simulink model "test55"  (R2015a)
settings: Solver=ode4  StartTime=0.0  StopTime=10  FixedStep=0.0001  RelTol=1e-3
values from neighbouring files (symbols this model uses):
  d1 = m0 + m1 + m2    (= 2.75)    [test3.m]    (also in test4.m; test5.m = 0.00498784618394)
  d2 = (m1/2 + m2) * l1    (= 0.5)    [test3.m]    (also in test4.m; test5.m = 0.00670234055869)
  d3 = m2 * l2/2    (= 0.28125)    [test3.m]    (also in test4.m; test5.m = 0.00902586221044)
  f1 = (m1/2 + m2) * l1 * g    (= 4.9)    [test3.m]    (also in test4.m; test5.m = 0.66350669926)
  f2 = m2 * l2 *g/2    (= 2.75625)    [test3.m]    (also in test4.m; test5.m = 0.891162386564)
settings Model: Creator=joseg  LastModifiedBy=joseg
settings SolverCC: AlgebraicLoopSolver=LineSearch

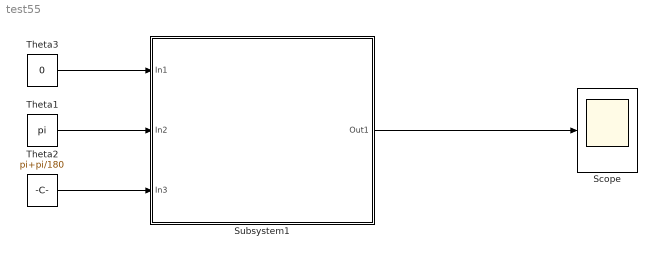
== system test55 ==
  Scope : Scope
      settings: TimeRange=14.3  YMin=-40000  YMax=5000
  Subsystem1 : Subsystem
  Theta1 : Constant  Value=pi
  Theta2 : Constant  Value=pi+pi/180
  Theta3 : Constant  Value=0
  wires:
  Theta1/1 -> Subsystem1/2(In2)
  Theta2/1 -> Subsystem1/3(In3)
  Theta3/1 -> Subsystem1/1(In1)
  Subsystem1/1(Out1) -> Scope/1

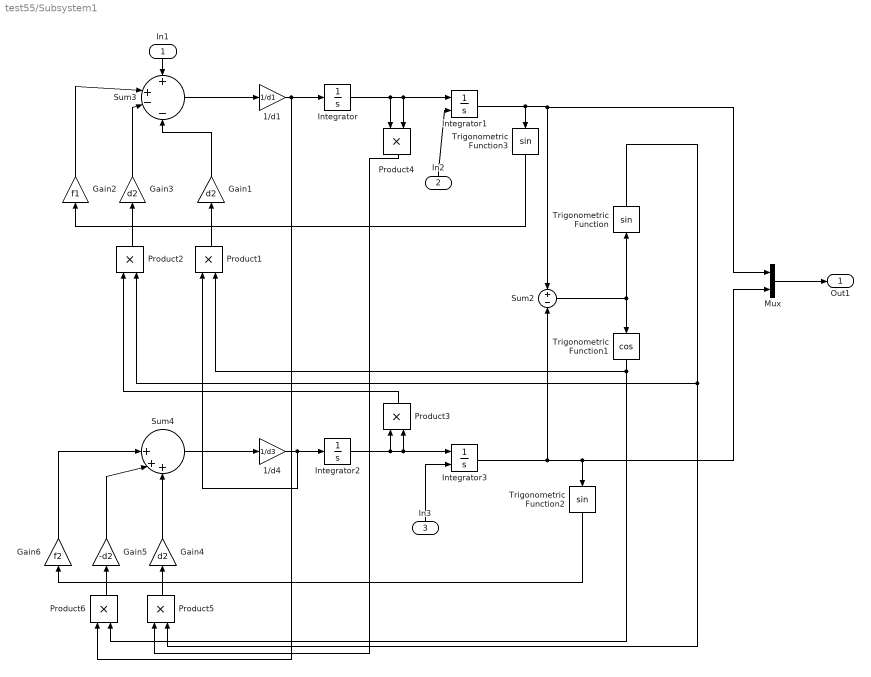
== system test55/Subsystem1 ==
  In1 : Inport
  In2 : Inport  Port=2
  In3 : Inport  Port=3
  1/d1 : Gain  Gain=1/d1
  1/d4 : Gain  Gain=1/d3
  Gain1 : Gain  Gain=d2
  Gain2 : Gain  Gain=f1
  Gain3 : Gain  Gain=d2
  Gain4 : Gain  Gain=d2
  Gain5 : Gain  Gain=-d2
  Gain6 : Gain  Gain=f2
  Integrator : Integrator
  Integrator1 : Integrator  InitialConditionSource=external
  Integrator2 : Integrator
  Integrator3 : Integrator  InitialConditionSource=external
  Mux : Mux  Inputs=2
  Product{1..6} (6 alike) : Product
  Sum2 : Sum  Inputs=+|-
  Sum3 : Sum  Inputs=+|+-|-
  Sum4 : Sum  Inputs=||+++
  Trigonometric Function : Trigonometry
  Trigonometric Function1 : Trigonometry  Operator=cos
  Trigonometric Function2 : Trigonometry
  Trigonometric Function3 : Trigonometry
  Out1 : Outport
  wires:
  Trigonometric Function/1 -> Product5/2, Product2/2
  Integrator2/1 -> Integrator3/1, Product3/2, Product3/1
  Product3/1 -> Product2/1
  Product6/1 -> Gain5/1
  Integrator/1 -> Product4/1, Product4/2, Integrator1/1
  Product5/1 -> Gain4/1
  Gain5/1 -> Sum4/2
  Trigonometric Function3/1 -> Gain2/1
  Gain4/1 -> Sum4/3
  Trigonometric Function1/1 -> Product6/2, Product1/2
  1/d4/1 -> Integrator2/1, Product1/1
  Product4/1 -> Product5/1
  Product2/1 -> Gain3/1
  In1/1 -> Sum3/1
  Gain6/1 -> Sum4/1
  Product1/1 -> Gain1/1
  Gain2/1 -> Sum3/2
  Gain1/1 -> Sum3/4
  Trigonometric Function2/1 -> Gain6/1
  Sum4/1 -> 1/d4/1
  1/d1/1 -> Integrator/1, Product6/1
  Sum3/1 -> 1/d1/1
  Integrator3/1 -> Trigonometric Function2/1, Mux/2, Sum2/2
  Sum2/1 -> Trigonometric Function1/1, Trigonometric Function/1
  Integrator1/1 -> Trigonometric Function3/1, Mux/1, Sum2/1
  Gain3/1 -> Sum3/3
  In2/1 -> Integrator1/2
  In3/1 -> Integrator3/2
  Mux/1 -> Out1/1
